simulink model "g1_opam_step_01"  (R2025b)
settings: Solver=ode1  StartTime=0.0  StopTime=Inf  FixedStep=Ts  RelTol=1e-3
PostLoadFcn:
  | GL_cbfcn('PostLoadFcn');
InitFcn:
  | GL_cbfcn('InitFcn');
StartFcn:
  | GL_cbfcn('StartFcn');
undefined symbols (not defined in the file or in its folder): burblks, DiscIntNeverNeededParam
libraries: bur_blks x1
(part 2 of 2)

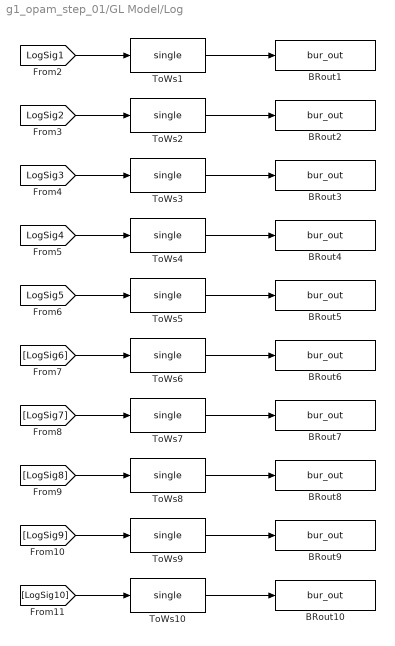
== system g1_opam_step_01/GL Model/Log ==
  BRout1 : S-Function  Tag=GLOBAL REAL rSimLogVar1  Description=burblks.classes.blks.BR_OutputBlock.Do('open', gcb)  LoadFcn=burblks.classes.blks.BR_OutputBlock.Do( 'load', gcb)  InitFcn=burblks.classes.blks.BR_OutputBlock.Do('init', gcb)  FunctionName=bur_out  Parameters=bur_scope, bur_data_type, bur_init_value, bur_init_value_bool, bur_array_index, bur_var_name, bur_AS_string  SFunctionDeploymentMode=off  EnableBusSupport=off  mask(B&&R - Output Block){bur_var_name=rSimLogVar1, bur_var_description=, bur_scope=GLOBAL, bur_data_type=REAL, bur_init_value=0, bur_init_value_bool=FALSE, bur_array_index=0, bur_old_var_name=, bur_var_memory=standard, bur_AS_string=rSimLogVar1 : REAL := 0; (**), bur_array_index_string=0}
      mask prompts: bur_var_name "Variable Name"; bur_var_description "Variable Description"; bur_scope "Variable Scope"; bur_data_type "Variable Data Type"; bur_init_value "Initial Value"; bur_init_value_bool "Initial Value"; bur_array_index "Array Dimension (0...Scalar)"; bur_old_var_name "Old Variable Name"; bur_var_memory "Memory"; bur_array_index_string "Array Dimension Variable (0..Scalar)"
      mask help: Output interface for B&R Automation Studio process variable.
      settings: AttributesFormatString=%<Tag>  CopyFcn=burblks.classes.blks.BR_OutputBlock.Do('copy', gcb)  DeleteFcn=burblks.classes.blks.BR_OutputBlock.Do( 'delete', gcb)  ModelCloseFcn=burblks.classes.blks.BR_OutputBlock.Do('close', gcb)  PreSaveFcn=burblks.classes.blks.BR_OutputBlock.Do('preSave', gcb)  PostSaveFcn=burblks.classes.blks.BR_OutputBlock.Do('postSave', gcb)  OpenFcn=burblks.classes.blks.BR_OutputBlock.Do('open', gcb)
      mask Help: eval('burblks.classes.blks.BR_BlockHelp.Help(''OutputBlock'')')
      mask TypeOptions bur_scope: GLOBAL | LOCAL
      mask TypeOptions bur_data_type: LREAL | REAL | SINT | USINT | INT | UINT | DINT | UDINT | BOOL | STRING
      mask TypeOptions bur_init_value_bool: FALSE | TRUE
      mask TypeOptions bur_var_memory: standard | retain
      mask Display: color('orange'); disp('B&R OUT');
  BRout10 : S-Function  Tag=GLOBAL REAL rSimLogVar10  Description=burblks.classes.blks.BR_OutputBlock.Do('open', gcb)  LoadFcn=burblks.classes.blks.BR_OutputBlock.Do( 'load', gcb)  InitFcn=burblks.classes.blks.BR_OutputBlock.Do('init', gcb)  FunctionName=bur_out  Parameters=bur_scope, bur_data_type, bur_init_value, bur_init_value_bool, bur_array_index, bur_var_name, bur_AS_string  SFunctionDeploymentMode=off  EnableBusSupport=off  mask(B&&R - Output Block){bur_var_name=rSimLogVar10, bur_var_description=, bur_scope=GLOBAL, bur_data_type=REAL, bur_init_value=0, bur_init_value_bool=FALSE, bur_array_index=0, bur_old_var_name=, bur_var_memory=standard, bur_AS_string=rSimLogVar10 : REAL := 0; (**), bur_array_index_string=0}
      mask prompts: bur_var_name "Variable Name"; bur_var_description "Variable Description"; bur_scope "Variable Scope"; bur_data_type "Variable Data Type"; bur_init_value "Initial Value"; bur_init_value_bool "Initial Value"; bur_array_index "Array Dimension (0...Scalar)"; bur_old_var_name "Old Variable Name"; bur_var_memory "Memory"; bur_array_index_string "Array Dimension Variable (0..Scalar)"
      mask help: Output interface for B&R Automation Studio process variable.
      settings: AttributesFormatString=%<Tag>  CopyFcn=burblks.classes.blks.BR_OutputBlock.Do('copy', gcb)  DeleteFcn=burblks.classes.blks.BR_OutputBlock.Do( 'delete', gcb)  ModelCloseFcn=burblks.classes.blks.BR_OutputBlock.Do('close', gcb)  PreSaveFcn=burblks.classes.blks.BR_OutputBlock.Do('preSave', gcb)  PostSaveFcn=burblks.classes.blks.BR_OutputBlock.Do('postSave', gcb)  OpenFcn=burblks.classes.blks.BR_OutputBlock.Do('open', gcb)
      mask Help: eval('burblks.classes.blks.BR_BlockHelp.Help(''OutputBlock'')')
      mask TypeOptions bur_scope: GLOBAL | LOCAL
      mask TypeOptions bur_data_type: LREAL | REAL | SINT | USINT | INT | UINT | DINT | UDINT | BOOL | STRING
      mask TypeOptions bur_init_value_bool: FALSE | TRUE
      mask TypeOptions bur_var_memory: standard | retain
      mask Display: color('orange'); disp('B&R OUT');
  BRout2 : S-Function  Tag=GLOBAL REAL rSimLogVar2  Description=burblks.classes.blks.BR_OutputBlock.Do('open', gcb)  LoadFcn=burblks.classes.blks.BR_OutputBlock.Do( 'load', gcb)  InitFcn=burblks.classes.blks.BR_OutputBlock.Do('init', gcb)  FunctionName=bur_out  Parameters=bur_scope, bur_data_type, bur_init_value, bur_init_value_bool, bur_array_index, bur_var_name, bur_AS_string  SFunctionDeploymentMode=off  EnableBusSupport=off  mask(B&&R - Output Block){bur_var_name=rSimLogVar2, bur_var_description=, bur_scope=GLOBAL, bur_data_type=REAL, bur_init_value=0, bur_init_value_bool=FALSE, bur_array_index=0, bur_old_var_name=, bur_var_memory=standard, bur_AS_string=rSimLogVar2 : REAL := 0; (**), bur_array_index_string=0}
      mask prompts: bur_var_name "Variable Name"; bur_var_description "Variable Description"; bur_scope "Variable Scope"; bur_data_type "Variable Data Type"; bur_init_value "Initial Value"; bur_init_value_bool "Initial Value"; bur_array_index "Array Dimension (0...Scalar)"; bur_old_var_name "Old Variable Name"; bur_var_memory "Memory"; bur_array_index_string "Array Dimension Variable (0..Scalar)"
      mask help: Output interface for B&R Automation Studio process variable.
      settings: AttributesFormatString=%<Tag>  CopyFcn=burblks.classes.blks.BR_OutputBlock.Do('copy', gcb)  DeleteFcn=burblks.classes.blks.BR_OutputBlock.Do( 'delete', gcb)  ModelCloseFcn=burblks.classes.blks.BR_OutputBlock.Do('close', gcb)  PreSaveFcn=burblks.classes.blks.BR_OutputBlock.Do('preSave', gcb)  PostSaveFcn=burblks.classes.blks.BR_OutputBlock.Do('postSave', gcb)  OpenFcn=burblks.classes.blks.BR_OutputBlock.Do('open', gcb)
      mask Help: eval('burblks.classes.blks.BR_BlockHelp.Help(''OutputBlock'')')
      mask TypeOptions bur_scope: GLOBAL | LOCAL
      mask TypeOptions bur_data_type: LREAL | REAL | SINT | USINT | INT | UINT | DINT | UDINT | BOOL | STRING
      mask TypeOptions bur_init_value_bool: FALSE | TRUE
      mask TypeOptions bur_var_memory: standard | retain
      mask Display: color('orange'); disp('B&R OUT');
  BRout3 : S-Function  Tag=GLOBAL REAL rSimLogVar3  Description=burblks.classes.blks.BR_OutputBlock.Do('open', gcb)  LoadFcn=burblks.classes.blks.BR_OutputBlock.Do( 'load', gcb)  InitFcn=burblks.classes.blks.BR_OutputBlock.Do('init', gcb)  FunctionName=bur_out  Parameters=bur_scope, bur_data_type, bur_init_value, bur_init_value_bool, bur_array_index, bur_var_name, bur_AS_string  SFunctionDeploymentMode=off  EnableBusSupport=off  mask(B&&R - Output Block){bur_var_name=rSimLogVar3, bur_var_description=, bur_scope=GLOBAL, bur_data_type=REAL, bur_init_value=0, bur_init_value_bool=FALSE, bur_array_index=0, bur_old_var_name=, bur_var_memory=standard, bur_AS_string=rSimLogVar3 : REAL := 0; (**), bur_array_index_string=0}
      mask prompts: bur_var_name "Variable Name"; bur_var_description "Variable Description"; bur_scope "Variable Scope"; bur_data_type "Variable Data Type"; bur_init_value "Initial Value"; bur_init_value_bool "Initial Value"; bur_array_index "Array Dimension (0...Scalar)"; bur_old_var_name "Old Variable Name"; bur_var_memory "Memory"; bur_array_index_string "Array Dimension Variable (0..Scalar)"
      mask help: Output interface for B&R Automation Studio process variable.
      settings: AttributesFormatString=%<Tag>  CopyFcn=burblks.classes.blks.BR_OutputBlock.Do('copy', gcb)  DeleteFcn=burblks.classes.blks.BR_OutputBlock.Do( 'delete', gcb)  ModelCloseFcn=burblks.classes.blks.BR_OutputBlock.Do('close', gcb)  PreSaveFcn=burblks.classes.blks.BR_OutputBlock.Do('preSave', gcb)  PostSaveFcn=burblks.classes.blks.BR_OutputBlock.Do('postSave', gcb)  OpenFcn=burblks.classes.blks.BR_OutputBlock.Do('open', gcb)
      mask Help: eval('burblks.classes.blks.BR_BlockHelp.Help(''OutputBlock'')')
      mask TypeOptions bur_scope: GLOBAL | LOCAL
      mask TypeOptions bur_data_type: LREAL | REAL | SINT | USINT | INT | UINT | DINT | UDINT | BOOL | STRING
      mask TypeOptions bur_init_value_bool: FALSE | TRUE
      mask TypeOptions bur_var_memory: standard | retain
      mask Display: color('orange'); disp('B&R OUT');
  BRout4 : S-Function  Tag=GLOBAL REAL rSimLogVar4  Description=burblks.classes.blks.BR_OutputBlock.Do('open', gcb)  LoadFcn=burblks.classes.blks.BR_OutputBlock.Do( 'load', gcb)  InitFcn=burblks.classes.blks.BR_OutputBlock.Do('init', gcb)  FunctionName=bur_out  Parameters=bur_scope, bur_data_type, bur_init_value, bur_init_value_bool, bur_array_index, bur_var_name, bur_AS_string  SFunctionDeploymentMode=off  EnableBusSupport=off  mask(B&&R - Output Block){bur_var_name=rSimLogVar4, bur_var_description=, bur_scope=GLOBAL, bur_data_type=REAL, bur_init_value=0, bur_init_value_bool=FALSE, bur_array_index=0, bur_old_var_name=, bur_var_memory=standard, bur_AS_string=rSimLogVar4 : REAL := 0; (**), bur_array_index_string=0}
      mask prompts: bur_var_name "Variable Name"; bur_var_description "Variable Description"; bur_scope "Variable Scope"; bur_data_type "Variable Data Type"; bur_init_value "Initial Value"; bur_init_value_bool "Initial Value"; bur_array_index "Array Dimension (0...Scalar)"; bur_old_var_name "Old Variable Name"; bur_var_memory "Memory"; bur_array_index_string "Array Dimension Variable (0..Scalar)"
      mask help: Output interface for B&R Automation Studio process variable.
      settings: AttributesFormatString=%<Tag>  CopyFcn=burblks.classes.blks.BR_OutputBlock.Do('copy', gcb)  DeleteFcn=burblks.classes.blks.BR_OutputBlock.Do( 'delete', gcb)  ModelCloseFcn=burblks.classes.blks.BR_OutputBlock.Do('close', gcb)  PreSaveFcn=burblks.classes.blks.BR_OutputBlock.Do('preSave', gcb)  PostSaveFcn=burblks.classes.blks.BR_OutputBlock.Do('postSave', gcb)  OpenFcn=burblks.classes.blks.BR_OutputBlock.Do('open', gcb)
      mask Help: eval('burblks.classes.blks.BR_BlockHelp.Help(''OutputBlock'')')
      mask TypeOptions bur_scope: GLOBAL | LOCAL
      mask TypeOptions bur_data_type: LREAL | REAL | SINT | USINT | INT | UINT | DINT | UDINT | BOOL | STRING
      mask TypeOptions bur_init_value_bool: FALSE | TRUE
      mask TypeOptions bur_var_memory: standard | retain
      mask Display: color('orange'); disp('B&R OUT');
  BRout5 : S-Function  Tag=GLOBAL REAL rSimLogVar5  Description=burblks.classes.blks.BR_OutputBlock.Do('open', gcb)  LoadFcn=burblks.classes.blks.BR_OutputBlock.Do( 'load', gcb)  InitFcn=burblks.classes.blks.BR_OutputBlock.Do('init', gcb)  FunctionName=bur_out  Parameters=bur_scope, bur_data_type, bur_init_value, bur_init_value_bool, bur_array_index, bur_var_name, bur_AS_string  SFunctionDeploymentMode=off  EnableBusSupport=off  mask(B&&R - Output Block){bur_var_name=rSimLogVar5, bur_var_description=, bur_scope=GLOBAL, bur_data_type=REAL, bur_init_value=0, bur_init_value_bool=FALSE, bur_array_index=0, bur_old_var_name=, bur_var_memory=standard, bur_AS_string=rSimLogVar5 : REAL := 0; (**), bur_array_index_string=0}
      mask prompts: bur_var_name "Variable Name"; bur_var_description "Variable Description"; bur_scope "Variable Scope"; bur_data_type "Variable Data Type"; bur_init_value "Initial Value"; bur_init_value_bool "Initial Value"; bur_array_index "Array Dimension (0...Scalar)"; bur_old_var_name "Old Variable Name"; bur_var_memory "Memory"; bur_array_index_string "Array Dimension Variable (0..Scalar)"
      mask help: Output interface for B&R Automation Studio process variable.
      settings: AttributesFormatString=%<Tag>  CopyFcn=burblks.classes.blks.BR_OutputBlock.Do('copy', gcb)  DeleteFcn=burblks.classes.blks.BR_OutputBlock.Do( 'delete', gcb)  ModelCloseFcn=burblks.classes.blks.BR_OutputBlock.Do('close', gcb)  PreSaveFcn=burblks.classes.blks.BR_OutputBlock.Do('preSave', gcb)  PostSaveFcn=burblks.classes.blks.BR_OutputBlock.Do('postSave', gcb)  OpenFcn=burblks.classes.blks.BR_OutputBlock.Do('open', gcb)
      mask Help: eval('burblks.classes.blks.BR_BlockHelp.Help(''OutputBlock'')')
      mask TypeOptions bur_scope: GLOBAL | LOCAL
      mask TypeOptions bur_data_type: LREAL | REAL | SINT | USINT | INT | UINT | DINT | UDINT | BOOL | STRING
      mask TypeOptions bur_init_value_bool: FALSE | TRUE
      mask TypeOptions bur_var_memory: standard | retain
      mask Display: color('orange'); disp('B&R OUT');
  BRout6 : S-Function  Tag=GLOBAL REAL rSimLogVar6  Description=burblks.classes.blks.BR_OutputBlock.Do('open', gcb)  LoadFcn=burblks.classes.blks.BR_OutputBlock.Do( 'load', gcb)  InitFcn=burblks.classes.blks.BR_OutputBlock.Do('init', gcb)  FunctionName=bur_out  Parameters=bur_scope, bur_data_type, bur_init_value, bur_init_value_bool, bur_array_index, bur_var_name, bur_AS_string  SFunctionDeploymentMode=off  EnableBusSupport=off  mask(B&&R - Output Block){bur_var_name=rSimLogVar6, bur_var_description=, bur_scope=GLOBAL, bur_data_type=REAL, bur_init_value=0, bur_init_value_bool=FALSE, bur_array_index=0, bur_old_var_name=, bur_var_memory=standard, bur_AS_string=rSimLogVar6 : REAL := 0; (**), bur_array_index_string=0}
      mask prompts: bur_var_name "Variable Name"; bur_var_description "Variable Description"; bur_scope "Variable Scope"; bur_data_type "Variable Data Type"; bur_init_value "Initial Value"; bur_init_value_bool "Initial Value"; bur_array_index "Array Dimension (0...Scalar)"; bur_old_var_name "Old Variable Name"; bur_var_memory "Memory"; bur_array_index_string "Array Dimension Variable (0..Scalar)"
      mask help: Output interface for B&R Automation Studio process variable.
      settings: AttributesFormatString=%<Tag>  CopyFcn=burblks.classes.blks.BR_OutputBlock.Do('copy', gcb)  DeleteFcn=burblks.classes.blks.BR_OutputBlock.Do( 'delete', gcb)  ModelCloseFcn=burblks.classes.blks.BR_OutputBlock.Do('close', gcb)  PreSaveFcn=burblks.classes.blks.BR_OutputBlock.Do('preSave', gcb)  PostSaveFcn=burblks.classes.blks.BR_OutputBlock.Do('postSave', gcb)  OpenFcn=burblks.classes.blks.BR_OutputBlock.Do('open', gcb)
      mask Help: eval('burblks.classes.blks.BR_BlockHelp.Help(''OutputBlock'')')
      mask TypeOptions bur_scope: GLOBAL | LOCAL
      mask TypeOptions bur_data_type: LREAL | REAL | SINT | USINT | INT | UINT | DINT | UDINT | BOOL | STRING
      mask TypeOptions bur_init_value_bool: FALSE | TRUE
      mask TypeOptions bur_var_memory: standard | retain
      mask Display: color('orange'); disp('B&R OUT');
  BRout7 : S-Function  Tag=GLOBAL REAL rSimLogVar7  Description=burblks.classes.blks.BR_OutputBlock.Do('open', gcb)  LoadFcn=burblks.classes.blks.BR_OutputBlock.Do( 'load', gcb)  InitFcn=burblks.classes.blks.BR_OutputBlock.Do('init', gcb)  FunctionName=bur_out  Parameters=bur_scope, bur_data_type, bur_init_value, bur_init_value_bool, bur_array_index, bur_var_name, bur_AS_string  SFunctionDeploymentMode=off  EnableBusSupport=off  mask(B&&R - Output Block){bur_var_name=rSimLogVar7, bur_var_description=, bur_scope=GLOBAL, bur_data_type=REAL, bur_init_value=0, bur_init_value_bool=FALSE, bur_array_index=0, bur_old_var_name=, bur_var_memory=standard, bur_AS_string=rSimLogVar7 : REAL := 0; (**), bur_array_index_string=0}
      mask prompts: bur_var_name "Variable Name"; bur_var_description "Variable Description"; bur_scope "Variable Scope"; bur_data_type "Variable Data Type"; bur_init_value "Initial Value"; bur_init_value_bool "Initial Value"; bur_array_index "Array Dimension (0...Scalar)"; bur_old_var_name "Old Variable Name"; bur_var_memory "Memory"; bur_array_index_string "Array Dimension Variable (0..Scalar)"
      mask help: Output interface for B&R Automation Studio process variable.
      settings: AttributesFormatString=%<Tag>  CopyFcn=burblks.classes.blks.BR_OutputBlock.Do('copy', gcb)  DeleteFcn=burblks.classes.blks.BR_OutputBlock.Do( 'delete', gcb)  ModelCloseFcn=burblks.classes.blks.BR_OutputBlock.Do('close', gcb)  PreSaveFcn=burblks.classes.blks.BR_OutputBlock.Do('preSave', gcb)  PostSaveFcn=burblks.classes.blks.BR_OutputBlock.Do('postSave', gcb)  OpenFcn=burblks.classes.blks.BR_OutputBlock.Do('open', gcb)
      mask Help: eval('burblks.classes.blks.BR_BlockHelp.Help(''OutputBlock'')')
      mask TypeOptions bur_scope: GLOBAL | LOCAL
      mask TypeOptions bur_data_type: LREAL | REAL | SINT | USINT | INT | UINT | DINT | UDINT | BOOL | STRING
      mask TypeOptions bur_init_value_bool: FALSE | TRUE
      mask TypeOptions bur_var_memory: standard | retain
      mask Display: color('orange'); disp('B&R OUT');
  BRout8 : S-Function  Tag=GLOBAL REAL rSimLogVar8  Description=burblks.classes.blks.BR_OutputBlock.Do('open', gcb)  LoadFcn=burblks.classes.blks.BR_OutputBlock.Do( 'load', gcb)  InitFcn=burblks.classes.blks.BR_OutputBlock.Do('init', gcb)  FunctionName=bur_out  Parameters=bur_scope, bur_data_type, bur_init_value, bur_init_value_bool, bur_array_index, bur_var_name, bur_AS_string  SFunctionDeploymentMode=off  EnableBusSupport=off  mask(B&&R - Output Block){bur_var_name=rSimLogVar8, bur_var_description=, bur_scope=GLOBAL, bur_data_type=REAL, bur_init_value=0, bur_init_value_bool=FALSE, bur_array_index=0, bur_old_var_name=, bur_var_memory=standard, bur_AS_string=rSimLogVar8 : REAL := 0; (**), bur_array_index_string=0}
      mask prompts: bur_var_name "Variable Name"; bur_var_description "Variable Description"; bur_scope "Variable Scope"; bur_data_type "Variable Data Type"; bur_init_value "Initial Value"; bur_init_value_bool "Initial Value"; bur_array_index "Array Dimension (0...Scalar)"; bur_old_var_name "Old Variable Name"; bur_var_memory "Memory"; bur_array_index_string "Array Dimension Variable (0..Scalar)"
      mask help: Output interface for B&R Automation Studio process variable.
      settings: AttributesFormatString=%<Tag>  CopyFcn=burblks.classes.blks.BR_OutputBlock.Do('copy', gcb)  DeleteFcn=burblks.classes.blks.BR_OutputBlock.Do( 'delete', gcb)  ModelCloseFcn=burblks.classes.blks.BR_OutputBlock.Do('close', gcb)  PreSaveFcn=burblks.classes.blks.BR_OutputBlock.Do('preSave', gcb)  PostSaveFcn=burblks.classes.blks.BR_OutputBlock.Do('postSave', gcb)  OpenFcn=burblks.classes.blks.BR_OutputBlock.Do('open', gcb)
      mask Help: eval('burblks.classes.blks.BR_BlockHelp.Help(''OutputBlock'')')
      mask TypeOptions bur_scope: GLOBAL | LOCAL
      mask TypeOptions bur_data_type: LREAL | REAL | SINT | USINT | INT | UINT | DINT | UDINT | BOOL | STRING
      mask TypeOptions bur_init_value_bool: FALSE | TRUE
      mask TypeOptions bur_var_memory: standard | retain
      mask Display: color('orange'); disp('B&R OUT');
  BRout9 : S-Function  Tag=GLOBAL REAL rSimLogVar9  Description=burblks.classes.blks.BR_OutputBlock.Do('open', gcb)  LoadFcn=burblks.classes.blks.BR_OutputBlock.Do( 'load', gcb)  InitFcn=burblks.classes.blks.BR_OutputBlock.Do('init', gcb)  FunctionName=bur_out  Parameters=bur_scope, bur_data_type, bur_init_value, bur_init_value_bool, bur_array_index, bur_var_name, bur_AS_string  SFunctionDeploymentMode=off  EnableBusSupport=off  mask(B&&R - Output Block){bur_var_name=rSimLogVar9, bur_var_description=, bur_scope=GLOBAL, bur_data_type=REAL, bur_init_value=0, bur_init_value_bool=FALSE, bur_array_index=0, bur_old_var_name=, bur_var_memory=standard, bur_AS_string=rSimLogVar9 : REAL := 0; (**), bur_array_index_string=0}
      mask prompts: bur_var_name "Variable Name"; bur_var_description "Variable Description"; bur_scope "Variable Scope"; bur_data_type "Variable Data Type"; bur_init_value "Initial Value"; bur_init_value_bool "Initial Value"; bur_array_index "Array Dimension (0...Scalar)"; bur_old_var_name "Old Variable Name"; bur_var_memory "Memory"; bur_array_index_string "Array Dimension Variable (0..Scalar)"
      mask help: Output interface for B&R Automation Studio process variable.
      settings: AttributesFormatString=%<Tag>  CopyFcn=burblks.classes.blks.BR_OutputBlock.Do('copy', gcb)  DeleteFcn=burblks.classes.blks.BR_OutputBlock.Do( 'delete', gcb)  ModelCloseFcn=burblks.classes.blks.BR_OutputBlock.Do('close', gcb)  PreSaveFcn=burblks.classes.blks.BR_OutputBlock.Do('preSave', gcb)  PostSaveFcn=burblks.classes.blks.BR_OutputBlock.Do('postSave', gcb)  OpenFcn=burblks.classes.blks.BR_OutputBlock.Do('open', gcb)
      mask Help: eval('burblks.classes.blks.BR_BlockHelp.Help(''OutputBlock'')')
      mask TypeOptions bur_scope: GLOBAL | LOCAL
      mask TypeOptions bur_data_type: LREAL | REAL | SINT | USINT | INT | UINT | DINT | UDINT | BOOL | STRING
      mask TypeOptions bur_init_value_bool: FALSE | TRUE
      mask TypeOptions bur_var_memory: standard | retain
      mask Display: color('orange'); disp('B&R OUT');
  ToWs{1..10} (10 alike) : DataTypeConversion  OutDataTypeStr=single  SaturateOnIntegerOverflow=off  RndMeth=Floor
  wires:
  [LogSig4] -> ToWs4/1
  [LogSig7] -> ToWs7/1
  [LogSig3] -> ToWs3/1
  ToWs7/1 -> BRout7/1
  [LogSig5] -> ToWs5/1
  [LogSig2] -> ToWs2/1
  ToWs6/1 -> BRout6/1
  ToWs4/1 -> BRout4/1
  ToWs2/1 -> BRout2/1
  ToWs3/1 -> BRout3/1
  [LogSig10] -> ToWs10/1
  ToWs10/1 -> BRout10/1
  ToWs9/1 -> BRout9/1
  ToWs5/1 -> BRout5/1
  [LogSig1] -> ToWs1/1
  [LogSig8] -> ToWs8/1
  ToWs8/1 -> BRout8/1
  [LogSig9] -> ToWs9/1
  [LogSig6] -> ToWs6/1
  ToWs1/1 -> BRout1/1

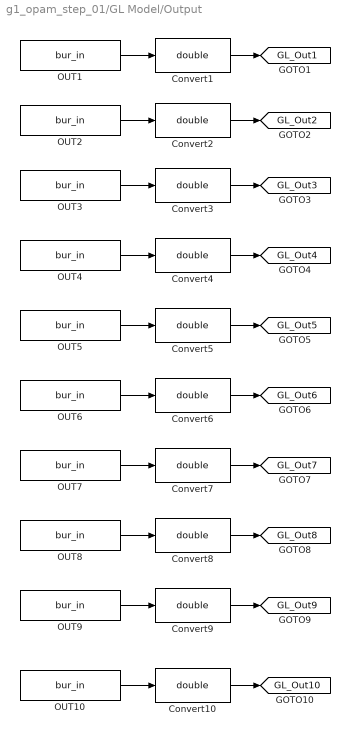
== system g1_opam_step_01/GL Model/Output ==
  Convert{1..10} (10 alike) : DataTypeConversion  OutDataTypeStr=double  SaturateOnIntegerOverflow=off  RndMeth=Floor
  OUT1 : S-Function  Tag=GLOBAL REAL rSimOutput1  Description=burblks.classes.blks.BR_InputBlock.Do('open', gcb)  LoadFcn=burblks.classes.blks.BR_InputBlock.Do( 'load', gcb)  InitFcn=burblks.classes.blks.BR_InputBlock.Do('init', gcb)  FunctionName=bur_in  Parameters=bur_scope, bur_data_type, bur_init_value, bur_init_value_bool, bur_array_index, bur_var_name, bur_AS_string  SFunctionDeploymentMode=off  EnableBusSupport=off  mask(B&&R - Input Block){bur_var_name=rSimOutput1, bur_var_description=, bur_scope=GLOBAL, bur_data_type=REAL, bur_init_value=0, bur_init_value_bool=FALSE, bur_array_index=0, bur_old_var_name=, bur_var_memory=standard, bur_in_parameter=off, bur_AS_string=rSimOutput1 : REAL := 0; (**), bur_array_index_string=0}
      mask prompts: bur_var_name "Variable Name"; bur_var_description "Variable Description"; bur_scope "Variable Scope"; bur_data_type "Variable Data Type"; bur_init_value "Initial Value"; bur_init_value_bool "Initial Value"; bur_array_index "Array Dimension (0...Scalar)"; bur_old_var_name "Old Variable Name"; bur_var_memory "Memory"; bur_in_parameter "Parameter"; bur_array_index_string "Array Dimension Variable (0..Scalar)"
      mask help: Input interface for B&R Automation Studio process variable.
      settings: AttributesFormatString=%<Tag>  CopyFcn=burblks.classes.blks.BR_InputBlock.Do('copy', gcb)  DeleteFcn=burblks.classes.blks.BR_InputBlock.Do( 'delete', gcb)  ModelCloseFcn=burblks.classes.blks.BR_InputBlock.Do('close', gcb)  PreSaveFcn=burblks.classes.blks.BR_InputBlock.Do('preSave', gcb)  PostSaveFcn=burblks.classes.blks.BR_InputBlock.Do('postSave', gcb)  OpenFcn=burblks.classes.blks.BR_InputBlock.Do('open', gcb)
      mask Help: eval('burblks.classes.blks.BR_BlockHelp.Help(''InputBlock'')')
      mask TypeOptions bur_scope: GLOBAL | LOCAL
      mask TypeOptions bur_data_type: LREAL | REAL | SINT | USINT | INT | UINT | DINT | UDINT | BOOL | STRING
      mask TypeOptions bur_init_value_bool: FALSE | TRUE
      mask TypeOptions bur_var_memory: standard | retain
      mask Display: color('orange'); disp('B&R IN');
  OUT10 : S-Function  Tag=GLOBAL REAL rSimOutput10  Description=burblks.classes.blks.BR_InputBlock.Do('open', gcb)  LoadFcn=burblks.classes.blks.BR_InputBlock.Do( 'load', gcb)  InitFcn=burblks.classes.blks.BR_InputBlock.Do('init', gcb)  FunctionName=bur_in  Parameters=bur_scope, bur_data_type, bur_init_value, bur_init_value_bool, bur_array_index, bur_var_name, bur_AS_string  SFunctionDeploymentMode=off  EnableBusSupport=off  mask(B&&R - Input Block){bur_var_name=rSimOutput10, bur_var_description=, bur_scope=GLOBAL, bur_data_type=REAL, bur_init_value=0, bur_init_value_bool=FALSE, bur_array_index=0, bur_old_var_name=, bur_var_memory=standard, bur_in_parameter=off, bur_AS_string=rSimOutput10 : REAL := 0; (**), bur_array_index_string=0}
      mask prompts: bur_var_name "Variable Name"; bur_var_description "Variable Description"; bur_scope "Variable Scope"; bur_data_type "Variable Data Type"; bur_init_value "Initial Value"; bur_init_value_bool "Initial Value"; bur_array_index "Array Dimension (0...Scalar)"; bur_old_var_name "Old Variable Name"; bur_var_memory "Memory"; bur_in_parameter "Parameter"; bur_array_index_string "Array Dimension Variable (0..Scalar)"
      mask help: Input interface for B&R Automation Studio process variable.
      settings: AttributesFormatString=%<Tag>  CopyFcn=burblks.classes.blks.BR_InputBlock.Do('copy', gcb)  DeleteFcn=burblks.classes.blks.BR_InputBlock.Do( 'delete', gcb)  ModelCloseFcn=burblks.classes.blks.BR_InputBlock.Do('close', gcb)  PreSaveFcn=burblks.classes.blks.BR_InputBlock.Do('preSave', gcb)  PostSaveFcn=burblks.classes.blks.BR_InputBlock.Do('postSave', gcb)  OpenFcn=burblks.classes.blks.BR_InputBlock.Do('open', gcb)
      mask Help: eval('burblks.classes.blks.BR_BlockHelp.Help(''InputBlock'')')
      mask TypeOptions bur_scope: GLOBAL | LOCAL
      mask TypeOptions bur_data_type: LREAL | REAL | SINT | USINT | INT | UINT | DINT | UDINT | BOOL | STRING
      mask TypeOptions bur_init_value_bool: FALSE | TRUE
      mask TypeOptions bur_var_memory: standard | retain
      mask Display: color('orange'); disp('B&R IN');
  OUT2 : S-Function  Tag=GLOBAL REAL rSimOutput2  Description=burblks.classes.blks.BR_InputBlock.Do('open', gcb)  LoadFcn=burblks.classes.blks.BR_InputBlock.Do( 'load', gcb)  InitFcn=burblks.classes.blks.BR_InputBlock.Do('init', gcb)  FunctionName=bur_in  Parameters=bur_scope, bur_data_type, bur_init_value, bur_init_value_bool, bur_array_index, bur_var_name, bur_AS_string  SFunctionDeploymentMode=off  EnableBusSupport=off  mask(B&&R - Input Block){bur_var_name=rSimOutput2, bur_var_description=, bur_scope=GLOBAL, bur_data_type=REAL, bur_init_value=0, bur_init_value_bool=FALSE, bur_array_index=0, bur_old_var_name=, bur_var_memory=standard, bur_in_parameter=off, bur_AS_string=rSimOutput2 : REAL := 0; (**), bur_array_index_string=0}
      mask prompts: bur_var_name "Variable Name"; bur_var_description "Variable Description"; bur_scope "Variable Scope"; bur_data_type "Variable Data Type"; bur_init_value "Initial Value"; bur_init_value_bool "Initial Value"; bur_array_index "Array Dimension (0...Scalar)"; bur_old_var_name "Old Variable Name"; bur_var_memory "Memory"; bur_in_parameter "Parameter"; bur_array_index_string "Array Dimension Variable (0..Scalar)"
      mask help: Input interface for B&R Automation Studio process variable.
      settings: AttributesFormatString=%<Tag>  CopyFcn=burblks.classes.blks.BR_InputBlock.Do('copy', gcb)  DeleteFcn=burblks.classes.blks.BR_InputBlock.Do( 'delete', gcb)  ModelCloseFcn=burblks.classes.blks.BR_InputBlock.Do('close', gcb)  PreSaveFcn=burblks.classes.blks.BR_InputBlock.Do('preSave', gcb)  PostSaveFcn=burblks.classes.blks.BR_InputBlock.Do('postSave', gcb)  OpenFcn=burblks.classes.blks.BR_InputBlock.Do('open', gcb)
      mask Help: eval('burblks.classes.blks.BR_BlockHelp.Help(''InputBlock'')')
      mask TypeOptions bur_scope: GLOBAL | LOCAL
      mask TypeOptions bur_data_type: LREAL | REAL | SINT | USINT | INT | UINT | DINT | UDINT | BOOL | STRING
      mask TypeOptions bur_init_value_bool: FALSE | TRUE
      mask TypeOptions bur_var_memory: standard | retain
      mask Display: color('orange'); disp('B&R IN');
  OUT3 : S-Function  Tag=GLOBAL REAL rSimOutput3  Description=burblks.classes.blks.BR_InputBlock.Do('open', gcb)  LoadFcn=burblks.classes.blks.BR_InputBlock.Do( 'load', gcb)  InitFcn=burblks.classes.blks.BR_InputBlock.Do('init', gcb)  FunctionName=bur_in  Parameters=bur_scope, bur_data_type, bur_init_value, bur_init_value_bool, bur_array_index, bur_var_name, bur_AS_string  SFunctionDeploymentMode=off  EnableBusSupport=off  mask(B&&R - Input Block){bur_var_name=rSimOutput3, bur_var_description=, bur_scope=GLOBAL, bur_data_type=REAL, bur_init_value=0, bur_init_value_bool=FALSE, bur_array_index=0, bur_old_var_name=, bur_var_memory=standard, bur_in_parameter=off, bur_AS_string=rSimOutput3 : REAL := 0; (**), bur_array_index_string=0}
      mask prompts: bur_var_name "Variable Name"; bur_var_description "Variable Description"; bur_scope "Variable Scope"; bur_data_type "Variable Data Type"; bur_init_value "Initial Value"; bur_init_value_bool "Initial Value"; bur_array_index "Array Dimension (0...Scalar)"; bur_old_var_name "Old Variable Name"; bur_var_memory "Memory"; bur_in_parameter "Parameter"; bur_array_index_string "Array Dimension Variable (0..Scalar)"
      mask help: Input interface for B&R Automation Studio process variable.
      settings: AttributesFormatString=%<Tag>  CopyFcn=burblks.classes.blks.BR_InputBlock.Do('copy', gcb)  DeleteFcn=burblks.classes.blks.BR_InputBlock.Do( 'delete', gcb)  ModelCloseFcn=burblks.classes.blks.BR_InputBlock.Do('close', gcb)  PreSaveFcn=burblks.classes.blks.BR_InputBlock.Do('preSave', gcb)  PostSaveFcn=burblks.classes.blks.BR_InputBlock.Do('postSave', gcb)  OpenFcn=burblks.classes.blks.BR_InputBlock.Do('open', gcb)
      mask Help: eval('burblks.classes.blks.BR_BlockHelp.Help(''InputBlock'')')
      mask TypeOptions bur_scope: GLOBAL | LOCAL
      mask TypeOptions bur_data_type: LREAL | REAL | SINT | USINT | INT | UINT | DINT | UDINT | BOOL | STRING
      mask TypeOptions bur_init_value_bool: FALSE | TRUE
      mask TypeOptions bur_var_memory: standard | retain
      mask Display: color('orange'); disp('B&R IN');
  OUT4 : S-Function  Tag=GLOBAL REAL rSimOutput4  Description=burblks.classes.blks.BR_InputBlock.Do('open', gcb)  LoadFcn=burblks.classes.blks.BR_InputBlock.Do( 'load', gcb)  InitFcn=burblks.classes.blks.BR_InputBlock.Do('init', gcb)  FunctionName=bur_in  Parameters=bur_scope, bur_data_type, bur_init_value, bur_init_value_bool, bur_array_index, bur_var_name, bur_AS_string  SFunctionDeploymentMode=off  EnableBusSupport=off  mask(B&&R - Input Block){bur_var_name=rSimOutput4, bur_var_description=, bur_scope=GLOBAL, bur_data_type=REAL, bur_init_value=0, bur_init_value_bool=FALSE, bur_array_index=0, bur_old_var_name=, bur_var_memory=standard, bur_in_parameter=off, bur_AS_string=rSimOutput4 : REAL := 0; (**), bur_array_index_string=0}
      mask prompts: bur_var_name "Variable Name"; bur_var_description "Variable Description"; bur_scope "Variable Scope"; bur_data_type "Variable Data Type"; bur_init_value "Initial Value"; bur_init_value_bool "Initial Value"; bur_array_index "Array Dimension (0...Scalar)"; bur_old_var_name "Old Variable Name"; bur_var_memory "Memory"; bur_in_parameter "Parameter"; bur_array_index_string "Array Dimension Variable (0..Scalar)"
      mask help: Input interface for B&R Automation Studio process variable.
      settings: AttributesFormatString=%<Tag>  CopyFcn=burblks.classes.blks.BR_InputBlock.Do('copy', gcb)  DeleteFcn=burblks.classes.blks.BR_InputBlock.Do( 'delete', gcb)  ModelCloseFcn=burblks.classes.blks.BR_InputBlock.Do('close', gcb)  PreSaveFcn=burblks.classes.blks.BR_InputBlock.Do('preSave', gcb)  PostSaveFcn=burblks.classes.blks.BR_InputBlock.Do('postSave', gcb)  OpenFcn=burblks.classes.blks.BR_InputBlock.Do('open', gcb)
      mask Help: eval('burblks.classes.blks.BR_BlockHelp.Help(''InputBlock'')')
      mask TypeOptions bur_scope: GLOBAL | LOCAL
      mask TypeOptions bur_data_type: LREAL | REAL | SINT | USINT | INT | UINT | DINT | UDINT | BOOL | STRING
      mask TypeOptions bur_init_value_bool: FALSE | TRUE
      mask TypeOptions bur_var_memory: standard | retain
      mask Display: color('orange'); disp('B&R IN');
  OUT5 : S-Function  Tag=GLOBAL BOOL rSimOutput5  Description=burblks.classes.blks.BR_InputBlock.Do('open', gcb)  LoadFcn=burblks.classes.blks.BR_InputBlock.Do( 'load', gcb)  InitFcn=burblks.classes.blks.BR_InputBlock.Do('init', gcb)  FunctionName=bur_in  Parameters=bur_scope, bur_data_type, bur_init_value, bur_init_value_bool, bur_array_index, bur_var_name, bur_AS_string  SFunctionDeploymentMode=off  EnableBusSupport=off  mask(B&&R - Input Block){bur_var_name=rSimOutput5, bur_var_description=, bur_scope=GLOBAL, bur_data_type=BOOL, bur_init_value=0, bur_init_value_bool=FALSE, bur_array_index=0, bur_old_var_name=, bur_var_memory=standard, bur_in_parameter=off, bur_AS_string=rSimOutput5 : BOOL := 0; (**), bur_array_index_string=0}
      mask prompts: bur_var_name "Variable Name"; bur_var_description "Variable Description"; bur_scope "Variable Scope"; bur_data_type "Variable Data Type"; bur_init_value "Initial Value"; bur_init_value_bool "Initial Value"; bur_array_index "Array Dimension (0...Scalar)"; bur_old_var_name "Old Variable Name"; bur_var_memory "Memory"; bur_in_parameter "Parameter"; bur_array_index_string "Array Dimension Variable (0..Scalar)"
      mask help: Input interface for B&R Automation Studio process variable.
      settings: AttributesFormatString=%<Tag>  CopyFcn=burblks.classes.blks.BR_InputBlock.Do('copy', gcb)  DeleteFcn=burblks.classes.blks.BR_InputBlock.Do( 'delete', gcb)  ModelCloseFcn=burblks.classes.blks.BR_InputBlock.Do('close', gcb)  PreSaveFcn=burblks.classes.blks.BR_InputBlock.Do('preSave', gcb)  PostSaveFcn=burblks.classes.blks.BR_InputBlock.Do('postSave', gcb)  OpenFcn=burblks.classes.blks.BR_InputBlock.Do('open', gcb)
      mask Help: eval('burblks.classes.blks.BR_BlockHelp.Help(''InputBlock'')')
      mask TypeOptions bur_scope: GLOBAL | LOCAL
      mask TypeOptions bur_data_type: LREAL | REAL | SINT | USINT | INT | UINT | DINT | UDINT | BOOL | STRING
      mask TypeOptions bur_init_value_bool: FALSE | TRUE
      mask TypeOptions bur_var_memory: standard | retain
      mask Display: color('orange'); disp('B&R IN');
  OUT6 : S-Function  Tag=GLOBAL REAL rSimOutput6  Description=burblks.classes.blks.BR_InputBlock.Do('open', gcb)  LoadFcn=burblks.classes.blks.BR_InputBlock.Do( 'load', gcb)  InitFcn=burblks.classes.blks.BR_InputBlock.Do('init', gcb)  FunctionName=bur_in  Parameters=bur_scope, bur_data_type, bur_init_value, bur_init_value_bool, bur_array_index, bur_var_name, bur_AS_string  SFunctionDeploymentMode=off  EnableBusSupport=off  mask(B&&R - Input Block){bur_var_name=rSimOutput6, bur_var_description=, bur_scope=GLOBAL, bur_data_type=REAL, bur_init_value=0, bur_init_value_bool=FALSE, bur_array_index=0, bur_old_var_name=, bur_var_memory=standard, bur_in_parameter=off, bur_AS_string=rSimOutput6 : REAL := 0; (**), bur_array_index_string=0}
      mask prompts: bur_var_name "Variable Name"; bur_var_description "Variable Description"; bur_scope "Variable Scope"; bur_data_type "Variable Data Type"; bur_init_value "Initial Value"; bur_init_value_bool "Initial Value"; bur_array_index "Array Dimension (0...Scalar)"; bur_old_var_name "Old Variable Name"; bur_var_memory "Memory"; bur_in_parameter "Parameter"; bur_array_index_string "Array Dimension Variable (0..Scalar)"
      mask help: Input interface for B&R Automation Studio process variable.
      settings: AttributesFormatString=%<Tag>  CopyFcn=burblks.classes.blks.BR_InputBlock.Do('copy', gcb)  DeleteFcn=burblks.classes.blks.BR_InputBlock.Do( 'delete', gcb)  ModelCloseFcn=burblks.classes.blks.BR_InputBlock.Do('close', gcb)  PreSaveFcn=burblks.classes.blks.BR_InputBlock.Do('preSave', gcb)  PostSaveFcn=burblks.classes.blks.BR_InputBlock.Do('postSave', gcb)  OpenFcn=burblks.classes.blks.BR_InputBlock.Do('open', gcb)
      mask Help: eval('burblks.classes.blks.BR_BlockHelp.Help(''InputBlock'')')
      mask TypeOptions bur_scope: GLOBAL | LOCAL
      mask TypeOptions bur_data_type: LREAL | REAL | SINT | USINT | INT | UINT | DINT | UDINT | BOOL | STRING
      mask TypeOptions bur_init_value_bool: FALSE | TRUE
      mask TypeOptions bur_var_memory: standard | retain
      mask Display: color('orange'); disp('B&R IN');
  OUT7 : S-Function  Tag=GLOBAL REAL rSimOutput7  Description=burblks.classes.blks.BR_InputBlock.Do('open', gcb)  LoadFcn=burblks.classes.blks.BR_InputBlock.Do( 'load', gcb)  InitFcn=burblks.classes.blks.BR_InputBlock.Do('init', gcb)  FunctionName=bur_in  Parameters=bur_scope, bur_data_type, bur_init_value, bur_init_value_bool, bur_array_index, bur_var_name, bur_AS_string  SFunctionDeploymentMode=off  EnableBusSupport=off  mask(B&&R - Input Block){bur_var_name=rSimOutput7, bur_var_description=, bur_scope=GLOBAL, bur_data_type=REAL, bur_init_value=0, bur_init_value_bool=FALSE, bur_array_index=0, bur_old_var_name=, bur_var_memory=standard, bur_in_parameter=off, bur_AS_string=rSimOutput7 : REAL := 0; (**), bur_array_index_string=0}
      mask prompts: bur_var_name "Variable Name"; bur_var_description "Variable Description"; bur_scope "Variable Scope"; bur_data_type "Variable Data Type"; bur_init_value "Initial Value"; bur_init_value_bool "Initial Value"; bur_array_index "Array Dimension (0...Scalar)"; bur_old_var_name "Old Variable Name"; bur_var_memory "Memory"; bur_in_parameter "Parameter"; bur_array_index_string "Array Dimension Variable (0..Scalar)"
      mask help: Input interface for B&R Automation Studio process variable.
      settings: AttributesFormatString=%<Tag>  CopyFcn=burblks.classes.blks.BR_InputBlock.Do('copy', gcb)  DeleteFcn=burblks.classes.blks.BR_InputBlock.Do( 'delete', gcb)  ModelCloseFcn=burblks.classes.blks.BR_InputBlock.Do('close', gcb)  PreSaveFcn=burblks.classes.blks.BR_InputBlock.Do('preSave', gcb)  PostSaveFcn=burblks.classes.blks.BR_InputBlock.Do('postSave', gcb)  OpenFcn=burblks.classes.blks.BR_InputBlock.Do('open', gcb)
      mask Help: eval('burblks.classes.blks.BR_BlockHelp.Help(''InputBlock'')')
      mask TypeOptions bur_scope: GLOBAL | LOCAL
      mask TypeOptions bur_data_type: LREAL | REAL | SINT | USINT | INT | UINT | DINT | UDINT | BOOL | STRING
      mask TypeOptions bur_init_value_bool: FALSE | TRUE
      mask TypeOptions bur_var_memory: standard | retain
      mask Display: color('orange'); disp('B&R IN');
  OUT8 : S-Function  Tag=GLOBAL REAL rSimOutput8  Description=burblks.classes.blks.BR_InputBlock.Do('open', gcb)  LoadFcn=burblks.classes.blks.BR_InputBlock.Do( 'load', gcb)  InitFcn=burblks.classes.blks.BR_InputBlock.Do('init', gcb)  FunctionName=bur_in  Parameters=bur_scope, bur_data_type, bur_init_value, bur_init_value_bool, bur_array_index, bur_var_name, bur_AS_string  SFunctionDeploymentMode=off  EnableBusSupport=off  mask(B&&R - Input Block){bur_var_name=rSimOutput8, bur_var_description=, bur_scope=GLOBAL, bur_data_type=REAL, bur_init_value=0, bur_init_value_bool=FALSE, bur_array_index=0, bur_old_var_name=, bur_var_memory=standard, bur_in_parameter=off, bur_AS_string=rSimOutput8 : REAL := 0; (**), bur_array_index_string=0}
      mask prompts: bur_var_name "Variable Name"; bur_var_description "Variable Description"; bur_scope "Variable Scope"; bur_data_type "Variable Data Type"; bur_init_value "Initial Value"; bur_init_value_bool "Initial Value"; bur_array_index "Array Dimension (0...Scalar)"; bur_old_var_name "Old Variable Name"; bur_var_memory "Memory"; bur_in_parameter "Parameter"; bur_array_index_string "Array Dimension Variable (0..Scalar)"
      mask help: Input interface for B&R Automation Studio process variable.
      settings: AttributesFormatString=%<Tag>  CopyFcn=burblks.classes.blks.BR_InputBlock.Do('copy', gcb)  DeleteFcn=burblks.classes.blks.BR_InputBlock.Do( 'delete', gcb)  ModelCloseFcn=burblks.classes.blks.BR_InputBlock.Do('close', gcb)  PreSaveFcn=burblks.classes.blks.BR_InputBlock.Do('preSave', gcb)  PostSaveFcn=burblks.classes.blks.BR_InputBlock.Do('postSave', gcb)  OpenFcn=burblks.classes.blks.BR_InputBlock.Do('open', gcb)
      mask Help: eval('burblks.classes.blks.BR_BlockHelp.Help(''InputBlock'')')
      mask TypeOptions bur_scope: GLOBAL | LOCAL
      mask TypeOptions bur_data_type: LREAL | REAL | SINT | USINT | INT | UINT | DINT | UDINT | BOOL | STRING
      mask TypeOptions bur_init_value_bool: FALSE | TRUE
      mask TypeOptions bur_var_memory: standard | retain
      mask Display: color('orange'); disp('B&R IN');
  OUT9 : S-Function  Tag=GLOBAL REAL rSimOutput9  Description=burblks.classes.blks.BR_InputBlock.Do('open', gcb)  LoadFcn=burblks.classes.blks.BR_InputBlock.Do( 'load', gcb)  InitFcn=burblks.classes.blks.BR_InputBlock.Do('init', gcb)  FunctionName=bur_in  Parameters=bur_scope, bur_data_type, bur_init_value, bur_init_value_bool, bur_array_index, bur_var_name, bur_AS_string  SFunctionDeploymentMode=off  EnableBusSupport=off  mask(B&&R - Input Block){bur_var_name=rSimOutput9, bur_var_description=, bur_scope=GLOBAL, bur_data_type=REAL, bur_init_value=0, bur_init_value_bool=FALSE, bur_array_index=0, bur_old_var_name=, bur_var_memory=standard, bur_in_parameter=off, bur_AS_string=rSimOutput9 : REAL := 0; (**), bur_array_index_string=0}
      mask prompts: bur_var_name "Variable Name"; bur_var_description "Variable Description"; bur_scope "Variable Scope"; bur_data_type "Variable Data Type"; bur_init_value "Initial Value"; bur_init_value_bool "Initial Value"; bur_array_index "Array Dimension (0...Scalar)"; bur_old_var_name "Old Variable Name"; bur_var_memory "Memory"; bur_in_parameter "Parameter"; bur_array_index_string "Array Dimension Variable (0..Scalar)"
      mask help: Input interface for B&R Automation Studio process variable.
      settings: AttributesFormatString=%<Tag>  CopyFcn=burblks.classes.blks.BR_InputBlock.Do('copy', gcb)  DeleteFcn=burblks.classes.blks.BR_InputBlock.Do( 'delete', gcb)  ModelCloseFcn=burblks.classes.blks.BR_InputBlock.Do('close', gcb)  PreSaveFcn=burblks.classes.blks.BR_InputBlock.Do('preSave', gcb)  PostSaveFcn=burblks.classes.blks.BR_InputBlock.Do('postSave', gcb)  OpenFcn=burblks.classes.blks.BR_InputBlock.Do('open', gcb)
      mask Help: eval('burblks.classes.blks.BR_BlockHelp.Help(''InputBlock'')')
      mask TypeOptions bur_scope: GLOBAL | LOCAL
      mask TypeOptions bur_data_type: LREAL | REAL | SINT | USINT | INT | UINT | DINT | UDINT | BOOL | STRING
      mask TypeOptions bur_init_value_bool: FALSE | TRUE
      mask TypeOptions bur_var_memory: standard | retain
      mask Display: color('orange'); disp('B&R IN');
  tag scope: GL_Out10=global, GL_Out1=global, GL_Out2=global, GL_Out3=global, GL_Out4=global, GL_Out5=global, GL_Out6=global, GL_Out7=global, GL_Out8=global, GL_Out9=global
  wires:
  Convert10/1 -> [GL_Out10]
  Convert9/1 -> [GL_Out9]
  Convert8/1 -> [GL_Out8]
  Convert7/1 -> [GL_Out7]
  Convert6/1 -> [GL_Out6]
  Convert5/1 -> [GL_Out5]
  Convert4/1 -> [GL_Out4]
  Convert3/1 -> [GL_Out3]
  Convert2/1 -> [GL_Out2]
  Convert1/1 -> [GL_Out1]
  OUT1/1 -> Convert1/1
  OUT4/1 -> Convert4/1
  OUT2/1 -> Convert2/1
  OUT3/1 -> Convert3/1
  OUT5/1 -> Convert5/1
  OUT6/1 -> Convert6/1
  OUT7/1 -> Convert7/1
  OUT8/1 -> Convert8/1
  OUT9/1 -> Convert9/1
  OUT10/1 -> Convert10/1
